simulink library "btd"  (Simulink 8.1)
settings: Solver=ode1  StartTime=0.0  StopTime=Inf  FixedStep=0.001  RelTol=1e-3
PostLoadFcn:
  | , if any(exist('dsrtsu_mdlpostloadfcn', 'file') == [2, 3, 6]), try dsrtsu_mdlpostloadfcn('Execute', bdroot); catch fprintf('Error in PostLoadFcn (dsrtsu_mdlpostloadfcn) for model "%s":\n %s\n', bdroot, lasterr); end, end,
libraries: btnb x1, btb x1
settings Model: DSRTSU_INTERNAL_RTI_VER=450  DSRTSU_INTERNAL_RTI_TYPE=rti1401  RTICANMMDATA=struct('GeneralSetupData',struct('modelroot','D:\ELN150201_TAIWAN\trunk\AdasDragon\software\sw_development\arch\app\acc','generalsettings',struct('filesettings',struct('destfolder',struct('Name','RTICANMM_FILES','Check',1),'buildfolder',struct('Name','.','Check',1),'AbsDestfolder',struct('Name','D:\ELN150201_TAIWAN\trunk\AdasDragon\software\sw_development\arch\app\acc\RTICANMM_FILES'),'AbsBuildfolder',struct('Name','D:\ELN150201_TAIWAN\trunk\AdasDragon\software\sw_development\arch\app\acc'))),'options',struct('addpaths',1,'rmpaths',1,'addtrcexclusion',logical(1),'cannavigator',struct('checkmonitoring',0),'show_usrtrc',0,'use_usrtrc',0),'advanced',struct('options',[1 1 1 1 1 1 1 1 1 1 1 1 1 1 1 1 1 1 1 1 1 1 1 1 1 1 1 1 1 1 1 1 1 1 1 1 1 1 1 1 1 1 1 1 1 1 1 1 1 1 1 1 1 1 1 1 1 1 1 1 1 1 1 1 1 1 1 1 1 1 1 1 1 1 1 1 1 1 1 1 1 1 1 1 1 1 1 1 1 1 1 1 1 1 1 1 1 1 1 1]),'MPSetup',{{}},'modelname','btd','block','btd'))  DSRTSU_INTERNAL_RTIFPGA=40  Creator=AT015555  LastModifiedBy=AT015555

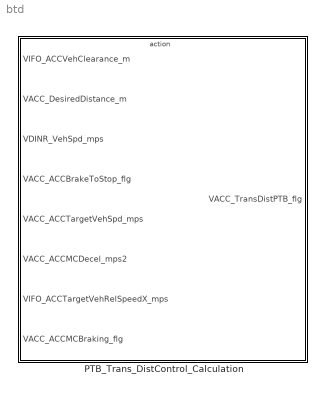
== system btd ==
  PTB_Trans_DistControl_Calculation : Subsystem  TreatAsAtomicUnit=on

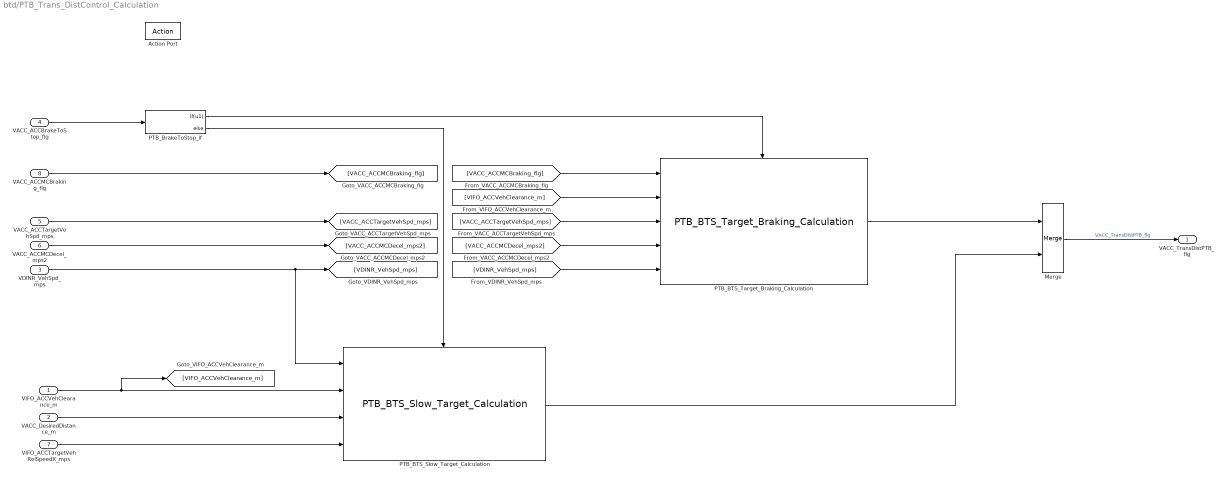
== system btd/PTB_Trans_DistControl_Calculation ==
  VIFO_ACCVehClearance_m : Inport
  VACC_DesiredDistance_m : Inport  Port=2
  VDINR_VehSpd_mps : Inport  Port=3
  VACC_ACCBrakeToStop_flg : Inport  Port=4
  VACC_ACCTargetVehSpd_mps : Inport  Port=5
  VACC_ACCMCDecel_mps2 : Inport  Port=6
  VIFO_ACCTargetVehRelSpeedX_mps : Inport  Port=7
  VACC_ACCMCBraking_flg : Inport  Port=8
  Action Port : ActionPort
  Merge : Merge
  PTB_BTS_Slow_Target_Calculation : btnb/PTB_BTS_Slow_Target_Calculation
  PTB_BTS_Target_Braking_Calculation : btb/PTB_BTS_Target_Braking_Calculation
  PTB_BrakeToStop_if : If  IfExpression=u1
  VACC_TransDistPTB_flg : Outport
  wires:
  VDINR_VehSpd_mps/1 -> PTB_BTS_Slow_Target_Calculation/1, [VDINR_VehSpd_mps]
  VACC_ACCBrakeToStop_flg/1 -> PTB_BrakeToStop_if/1
  PTB_BrakeToStop_if/1 -> PTB_BTS_Target_Braking_Calculation/Action
  PTB_BrakeToStop_if/2 -> PTB_BTS_Slow_Target_Calculation/Action
  VIFO_ACCVehClearance_m/1 -> PTB_BTS_Slow_Target_Calculation/2, [VIFO_ACCVehClearance_m]
  [VIFO_ACCVehClearance_m] -> PTB_BTS_Target_Braking_Calculation/2
  VACC_DesiredDistance_m/1 -> PTB_BTS_Slow_Target_Calculation/3
  VACC_ACCTargetVehSpd_mps/1 -> [VACC_ACCTargetVehSpd_mps]
  VACC_ACCMCDecel_mps2/1 -> [VACC_ACCMCDecel_mps2]
  VIFO_ACCTargetVehRelSpeedX_mps/1 -> PTB_BTS_Slow_Target_Calculation/4
  PTB_BTS_Target_Braking_Calculation/1 -> Merge/1
  PTB_BTS_Slow_Target_Calculation/1 -> Merge/2
  Merge/1 -> VACC_TransDistPTB_flg/1  "VACC_TransDistPTB_flg"
  VACC_ACCMCBraking_flg/1 -> [VACC_ACCMCBraking_flg]
  [VACC_ACCMCBraking_flg] -> PTB_BTS_Target_Braking_Calculation/1
  [VACC_ACCTargetVehSpd_mps] -> PTB_BTS_Target_Braking_Calculation/3
  [VACC_ACCMCDecel_mps2] -> PTB_BTS_Target_Braking_Calculation/4
  [VDINR_VehSpd_mps] -> PTB_BTS_Target_Braking_Calculation/5
